simulink model "propdraft"  (R2023b)
settings: Solver=VariableStepAuto  StartTime=0.0  StopTime=10.0  RelTol=1e-3
values from neighbouring files (symbols this model uses):
  dp_DEP =     [UNIFIER_LOAD.mat]    (also in UNIFIER_LOAD_ROM.mat)
  xyz_cg = [-8.09,0,-0.2]    [UNIFIER_LOAD.m]    (also in UNIFIER_LOAD.mat = [-8.09 0 -0.2]; UNIFIER_LOAD_ROM.m; UNIFIER_LOAD_ROM.mat = [-8.09 0 -0.2])
libraries: sharedutil x1, sharedtransform x1, simulink x1
settings Model: Creator=Reggie Johanes  LastModifiedBy=Reggie Johanes

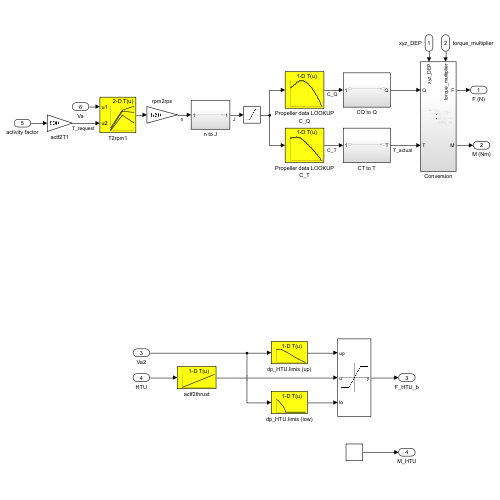
[thumbnail: Simulink's stored preview of the top-level diagram]
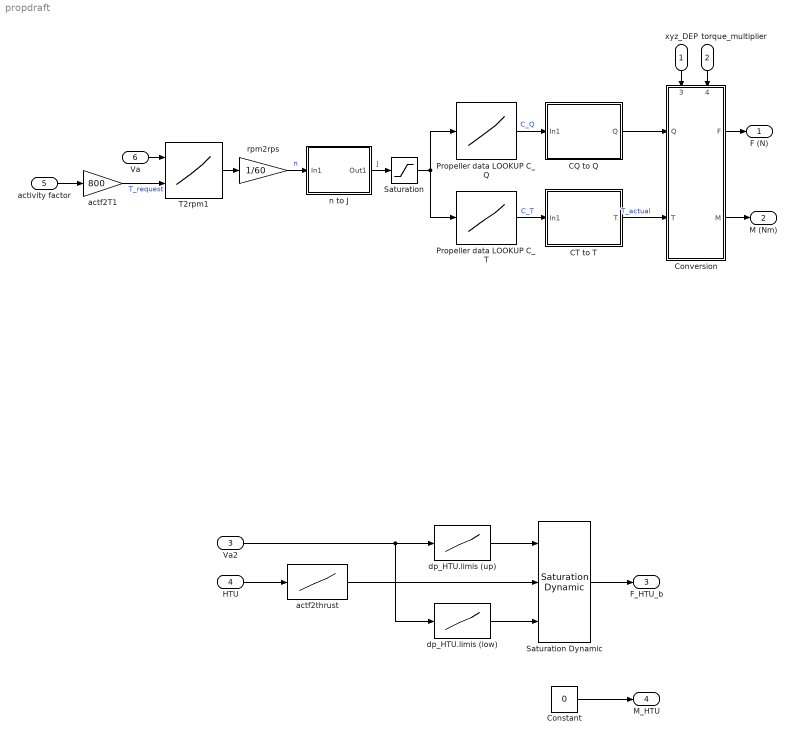
== system propdraft ==
  xyz_DEP : Inport
  torque_multiplier : Inport  Port=2
  Va2 : Inport  Port=3
  HTU : Inport  Port=4
  activity factor : Inport  Port=5
  Va : Inport  Port=6
  CQ to Q : Subsystem
  CT to T : Subsystem
  Constant : Constant  Value=0
  Conversion : Subsystem
      settings: PortSchema="{\"entries\":[{\"content\":{\"sides\":[{\"content\":{\"connectorIds\":[\"In1\",\"In2\"]},\"type\":\"ConnectorPlacement.EquallySpacedRectSide\",\"uuid\":\"e9c6c1f5-57bf-4dcc-bf48-2c7ecd161244\"},{\"content\":{\"connectorIds\":[\"Out1\",\"Out2\"],\"side\":\"RIGHT\"},\"type\":\"ConnectorPlacement.EquallySpacedRectSide\",\"uuid\":\"b5f2a1af-3b47-4f41-9c97-b4ecdcbd19d1\"},{\"content\":{\"connectorIds\":[\"In3\",\"In4\"],\"side\":\"TOP\"},\"type\":\"ConnectorPlacement.EquallySpacedRectSide\",\"uuid\":\"8f535440-cb03-4a3f-97c7-868271bf8893\"}]},\"type\":\"ConnectorPlacement.EquallySpacedConnector\",\"uuid\":\"e6936932-a2e3-496b-aaf7-92ca4c66a895\"}],\"packageUris\":[\"http://schema.mathworks.com/mf0/Connector/R2020b\"],\"version\":\"1.0\"}"
  Propeller data LOOKUP C_Q : Lookup_n-D  NumberOfTableDimensions=1  BreakpointsForDimension1=dp_DEP.J  IndexSearchMethod=Linear search  BeginIndexSearchUsingPreviousIndexResult=on  Table=dp_DEP.C_Q  ExtrapMethod=Clip  UseLastTableValue=on  InternalRulePriority=Speed  RndMeth=Simplest
  Propeller data LOOKUP C_T : Lookup_n-D  NumberOfTableDimensions=1  BreakpointsForDimension1=dp_DEP.J  IndexSearchMethod=Linear search  BeginIndexSearchUsingPreviousIndexResult=on  Table=dp_DEP.C_T  ExtrapMethod=Clip  UseLastTableValue=on  InternalRulePriority=Speed  RndMeth=Simplest
  Saturation : Saturate
  Saturation Dynamic : simulink/Discontinuities/Saturation Dynamic  OutMin=[]  OutMax=[]  OutDataTypeStr=Inherit: Same as second input  OutDataType=fixdt(1, 16)  OutScaling=2^-10  DoSatur=off
  T2rpm1 : Lookup_n-D  BreakpointsForDimension1=dp_DEP.rpm_lookup.V_vec  BreakpointsForDimension2=dp_DEP.rpm_lookup.T_vec  IndexSearchMethod=Linear search  BeginIndexSearchUsingPreviousIndexResult=on  Table=dp_DEP.rpm_lookup.rpm_gird  ExtrapMethod=Clip  InternalRulePriority=Speed  RndMeth=Simplest
      settings: InputPortMap=u0,u1
  actf2T1 : Gain  Gain=800
  actf2thrust : Lookup_n-D  NumberOfTableDimensions=1  BreakpointsForDimension1=[-0.5,1.5]  IndexSearchMethod=Linear search  BeginIndexSearchUsingPreviousIndexResult=on  Table=[-5000, 15000]  ExtrapMethod=Clip  InternalRulePriority=Speed  RndMeth=Simplest
  dp_HTU.limis (low) : Lookup_n-D  NumberOfTableDimensions=1  BreakpointsForDimension1=[20,25,30,35,40,80]  IndexSearchMethod=Linear search  BeginIndexSearchUsingPreviousIndexResult=on  Table=[-1000,-1500,-2500,-3500,-5000,-5000]  InternalRulePriority=Speed  RndMeth=Simplest
  dp_HTU.limis (up) : Lookup_n-D  NumberOfTableDimensions=1  BreakpointsForDimension1=[20,30,40,65,80]  IndexSearchMethod=Linear search  BeginIndexSearchUsingPreviousIndexResult=on  Table=[15000,15000,14000,11000,9500]  InternalRulePriority=Speed  RndMeth=Simplest
  n to J : Subsystem
  rpm2rps : Gain  Gain=1/60
  F (N) : Outport
  M (Nm) : Outport  Port=2
  F_HTU_b : Outport  Port=3
  M_HTU : Outport  Port=4
  wires:
  Conversion/1(F) -> F (N)/1
  Conversion/2(M) -> M (Nm)/1
  torque_multiplier/1 -> Conversion/4(torque_multiplier)
  rpm2rps/1 -> n to J/1(In1)  "n"
  CQ to Q/1(Q) -> Conversion/1(Q)
  CT to T/1(T) -> Conversion/2(T)  "T_actual"
  xyz_DEP/1 -> Conversion/3(xyz_DEP)
  Va2/1 -> dp_HTU.limis (low)/1, dp_HTU.limis (up)/1
  actf2thrust/1 -> Saturation Dynamic/2
  dp_HTU.limis (low)/1 -> Saturation Dynamic/3
  Saturation Dynamic/1 -> F_HTU_b/1
  Constant/1 -> M_HTU/1
  HTU/1 -> actf2thrust/1
  dp_HTU.limis (up)/1 -> Saturation Dynamic/1
  activity factor/1 -> actf2T1/1
  actf2T1/1 -> T2rpm1/2  "T_request"
  T2rpm1/1 -> rpm2rps/1
  Va/1 -> T2rpm1/1
  Propeller data LOOKUP C_T/1 -> CT to T/1(In1)  "C_T"
  Propeller data LOOKUP C_Q/1 -> CQ to Q/1(In1)  "C_Q"
  Saturation/1 -> Propeller data LOOKUP C_Q/1, Propeller data LOOKUP C_T/1
  n to J/1(Out1) -> Saturation/1  "J"

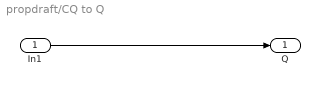
== system propdraft/CQ to Q ==
  In1 : Inport
  Q : Outport
  wires:
  In1/1 -> Q/1

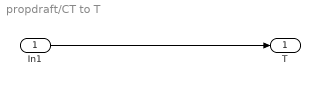
== system propdraft/CT to T ==
  In1 : Inport
  T : Outport
  wires:
  In1/1 -> T/1

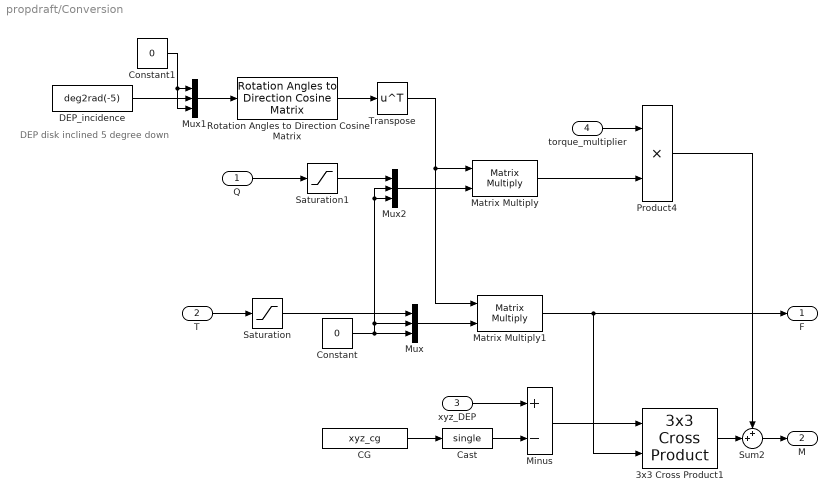
== system propdraft/Conversion ==
  note: DEP disk inclined 5 degree down
  Q : Inport
  T : Inport  Port=2
  xyz_DEP : Inport  Port=3
  torque_multiplier : Inport  Port=4
  3x3 Cross Product1 : sharedutil/3x3 Cross Product  aMode=aMode
  CG : Constant  Value=xyz_cg
  Cast : DataTypeConversion  OutDataTypeStr=single  SaturateOnIntegerOverflow=off  RndMeth=Floor
  Constant : Constant  Value=0
  Constant1 : Constant  Value=0
  DEP_incidence : Constant  Value=deg2rad(-5)
  Matrix Multiply : Product  Multiplication=Matrix(*)
  Matrix Multiply1 : Product  Multiplication=Matrix(*)
  Minus : Sum  Inputs=+-
  Mux : Mux  Inputs=3
  Mux1 : Mux  Inputs=3
  Mux2 : Mux  Inputs=3
  Product4 : Product
  Rotation Angles to Direction Cosine Matrix : sharedtransform/Rotation Angles to Direction Cosine Matrix  rotationOrder=ZYX  aMode=aMode
  Saturation : Saturate  UpperLimit=inf  LowerLimit=0
  Saturation1 : Saturate  UpperLimit=inf  LowerLimit=0
  Sum2 : Sum  Inputs=++|
  Transpose : Math  Operator=transpose
  F : Outport
  M : Outport  Port=2
  wires:
  Saturation1/1 -> Mux2/1
  T/1 -> Saturation/1
  Transpose/1 -> Matrix Multiply/1, Matrix Multiply1/1
  Q/1 -> Saturation1/1
  Constant/1 -> Mux/2, Mux2/2, Mux2/3, Mux/3
  Sum2/1 -> M/1
  Saturation/1 -> Mux/1
  3x3 Cross Product1/1 -> Sum2/2
  CG/1 -> Cast/1
  xyz_DEP/1 -> Minus/1
  Mux/1 -> Matrix Multiply1/2
  Mux1/1 -> Rotation Angles to Direction Cosine Matrix/1
  Minus/1 -> 3x3 Cross Product1/1
  Constant1/1 -> Mux1/1, Mux1/3
  Cast/1 -> Minus/2
  DEP_incidence/1 -> Mux1/2
  torque_multiplier/1 -> Product4/1
  Mux2/1 -> Matrix Multiply/2
  Matrix Multiply1/1 -> 3x3 Cross Product1/2, F/1
  Product4/1 -> Sum2/1
  Rotation Angles to Direction Cosine Matrix/1 -> Transpose/1
  Matrix Multiply/1 -> Product4/2

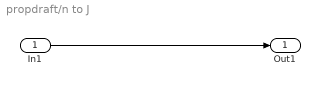
== system propdraft/n to J ==
  In1 : Inport
  Out1 : Outport
  wires:
  In1/1 -> Out1/1
